simulink model "system_identification_ssv"  (R2024b)
settings: Solver=VariableStepAuto  StartTime=0.0  StopTime=10  RelTol=1e-3
model workspace (MAT data in the model file):
  d = 0.5
  eps = 1
values from neighbouring files (symbols this model uses):
  s_L = slipRange(j)    [identify_system.m]
  s_R = slipRange(i)    [identify_system.m]
settings Model: Creator=radnor  LastModifiedBy=radnor

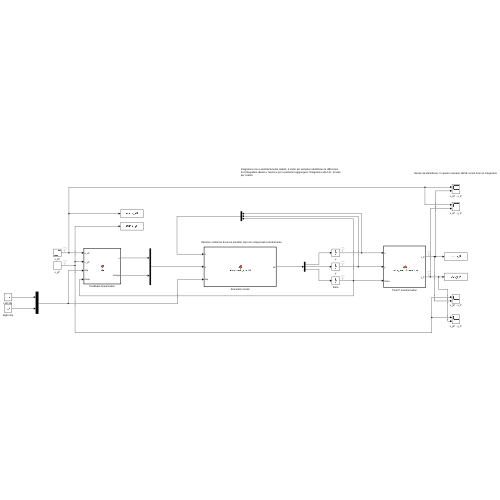
[thumbnail: Simulink's stored preview of the top-level diagram]
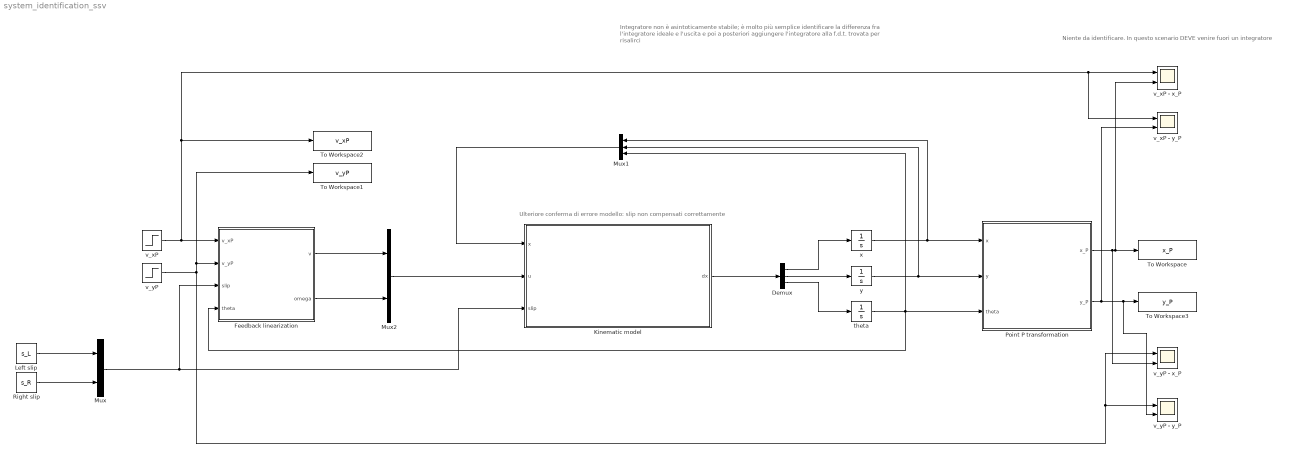
== system system_identification_ssv ==
  note: Integratore non è asintoticamente stabile; è molto più semplice identificare la differenza fra l'integratore ideale e l'uscita e poi a posteriori aggiungere l'integratore alla f.d.t. trovata per risalirci
  note: Niente da identificare. In questo scenario DEVE venire fuori un integratore
  note: Ulteriore conferma di errore modello: slip non compensati correttamente
  Demux : Demux  Outputs=3
  Feedback linearization : MATLAB Function  TreatAsAtomicUnit=on
  Kinematic model : MATLAB Function  TreatAsAtomicUnit=on
  Left slip : Constant  Value=s_L
  Mux : Mux  Inputs=2
  Mux1 : Mux  Inputs=3
  Mux2 : Mux  Inputs=2
  Point P transformation : MATLAB Function  TreatAsAtomicUnit=on
  Right slip : Constant  Value=s_R
  To Workspace : ToWorkspace  VariableName=x_P  SaveFormat=Timeseries  SampleTime=-1
  To Workspace1 : ToWorkspace  VariableName=v_yP  SaveFormat=Timeseries  SampleTime=-1
  To Workspace2 : ToWorkspace  VariableName=v_xP  SaveFormat=Timeseries  SampleTime=-1
  To Workspace3 : ToWorkspace  VariableName=y_P  SaveFormat=Timeseries  SampleTime=-1
  theta : Integrator
  v_xP : Step  Before=0.5  SampleTime=0
  v_xP - x_P : Scope  NumInputPorts=2
  v_xP - y_P : Scope  NumInputPorts=2
  v_yP : Step  Time=3  After=0.5  SampleTime=0
  v_yP - x_P : Scope  NumInputPorts=2
  v_yP - y_P : Scope  NumInputPorts=2
  x : Integrator
  y : Integrator
  wires:
  Mux/1 -> Feedback linearization/3(slip), Kinematic model/3(slip)
  Demux/1 -> x/1
  Demux/2 -> y/1
  Demux/3 -> theta/1
  Kinematic model/1(dx) -> Demux/1
  x/1 -> Point P transformation/1(x), Mux1/1
  y/1 -> Point P transformation/2(y), Mux1/2
  theta/1 -> Mux1/3, Point P transformation/3(theta), Feedback linearization/4(theta)
  Mux1/1 -> Kinematic model/1(x)
  Feedback linearization/1(v) -> Mux2/1
  Feedback linearization/2(omega) -> Mux2/2
  Mux2/1 -> Kinematic model/2(u)
  v_yP/1 -> To Workspace1/1, Feedback linearization/2(v_yP), v_yP - x_P/1, v_yP - y_P/1
  Point P transformation/1(x_P) -> v_yP - x_P/2, v_xP - x_P/2, To Workspace/1
  Point P transformation/2(y_P) -> v_yP - y_P/2, To Workspace3/1, v_xP - y_P/2
  Right slip/1 -> Mux/2
  Left slip/1 -> Mux/1
  v_xP/1 -> v_xP - y_P/1, v_xP - x_P/1, To Workspace2/1, Feedback linearization/1(v_xP)

== matlab function system_identification_ssv/Feedback linearization ==
  data: v_xP input; v output; v_yP input; slip input; theta input; omega output; eps parameter; d parameter
function [v, omega] = ssv(v_xP, v_yP, slip, theta, eps, d)
    eta_L = 1 - slip(1);
    eta_R = 1 - slip(2);
    gamma_11 = (eta_L + eta_R) / 2;
    gamma_12 = (eta_L - eta_R) / 2;
    gamma_21 = (eta_L + eta_R) / d;
    gamma_22 = (eta_L - eta_R) / d;

    a = (eps*gamma_11*cos(theta) - d*gamma_12*sin(theta)) / (eps*eta_R*eta_L);
    b = (eps*gamma_11*sin(theta) + d*gamma_12*cos(theta)) / (eps*eta_R*eta_L);
    c = (eps*gamma_22*cos(theta) - d*gamma_21*sin(theta)) / (eps*eta_R*eta_L);
    d = (eps*gamma_22*sin(theta) + d*gamma_21*cos(theta)) / (eps*eta_R*eta_L);

    v = a*v_xP + b*v_yP;
    omega = c*v_xP + d*v_yP;
end

== matlab function system_identification_ssv/Kinematic model ==
  data: x input size=3; u input; dx output size=3; slip input; d parameter
function dx = kinematic_model(x, u, slip, d)
    v = u(1);
    omega = u(2);

    theta = x(3);

    eta_L = 1-slip(1);
    eta_R = 1-slip(2);

    v_L = (v - d*omega) / eta_L;
    v_R = (v + d*omega) / eta_R;

    dx = zeros(3,1);
    dx(1) = 0.5*(eta_R*cos(theta)*v_R + eta_L*cos(theta)*v_L);
    dx(2) = 0.5*(eta_R*sin(theta)*v_R + eta_L*sin(theta)*v_L); 
    dx(3) = eta_R/(2*d)*v_R - eta_L/(2*d)*v_L;
end

== matlab function system_identification_ssv/Point P transformation ==
  data: x input; x_P output; y input; theta input; y_P output; eps parameter
function [x_P, y_P] = point_transformation(x, y, theta, eps)
    x_P = x + eps*cos(theta);
    y_P = y + eps*sin(theta);
end
